simulink model "Demo"  (R2024b)
settings: Solver=FixedStepDiscrete  StartTime=0.0  StopTime=15  FixedStep=0.001  RelTol=1e-3
InitFcn:
  | LCS_parameters
values from neighbouring files (symbols this model uses):
  BREFF = 1.9697    [LCS_parameters.m]
  carMass = 251.54    [LCS_parameters.m]
  CGheight = 0.253    [LCS_parameters.m]
  Cz = 87563    [LCS_parameters.m]
  DREFF = 0.54832    [LCS_parameters.m]
  FNOMIN = 1295    [LCS_parameters.m]
  FREFF = 0.017609    [LCS_parameters.m]
  gearRatio = 13.75    [LCS_parameters.m]
  LONGVL = 10    [LCS_parameters.m]
  nominalWheelRadius = 0.197    [LCS_parameters.m]
  optimalSlipRatio = 0.11    [LCS_parameters.m]
  Q_REO = 1    [LCS_parameters.m]
  Q_V1 = 0.0034187    [LCS_parameters.m]
  ss_error = [88.7600822305642	89.0376071734511	89.3159282635258	89.5955216735338	89.8756411218665	90.1570974487717	90.4395677327939	90.7230274541677	91.0072189085757	91.2921635447457	91.5779490537006	91.8650704841512	92.1538219996540	92.4426633861175	92.7316475908439	93.0233476422096	93.3140548464672	93.6068138765075	93.9008352694172	94.1935963586418	94.4902272246880	94.7850545124692	95.0823324329676	95.38056 ...(+2780 chars)    [LCS_parameters.m]
  unloadedRadius = 0.2032    [LCS_parameters.m]
  wheelbaseLength = 1.53    [LCS_parameters.m]
undefined symbols (not defined in the file or in its folder): dspblkCoreblockFVToolHelper, gcbh
libraries: Solver_SF x1, simulink x1
settings Model: NumberOfSteps=100  Creator=account  LastModifiedBy=xoxi.1

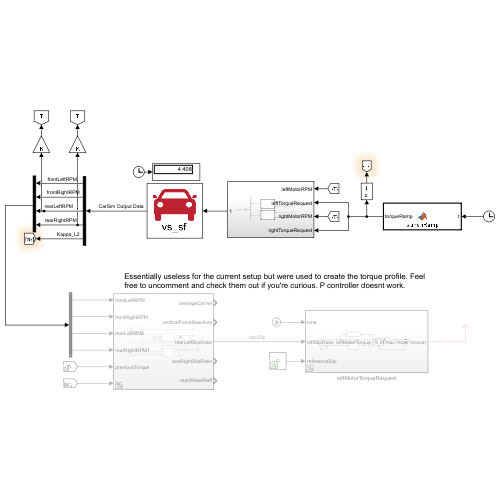
[thumbnail: Simulink's stored preview of the top-level diagram]
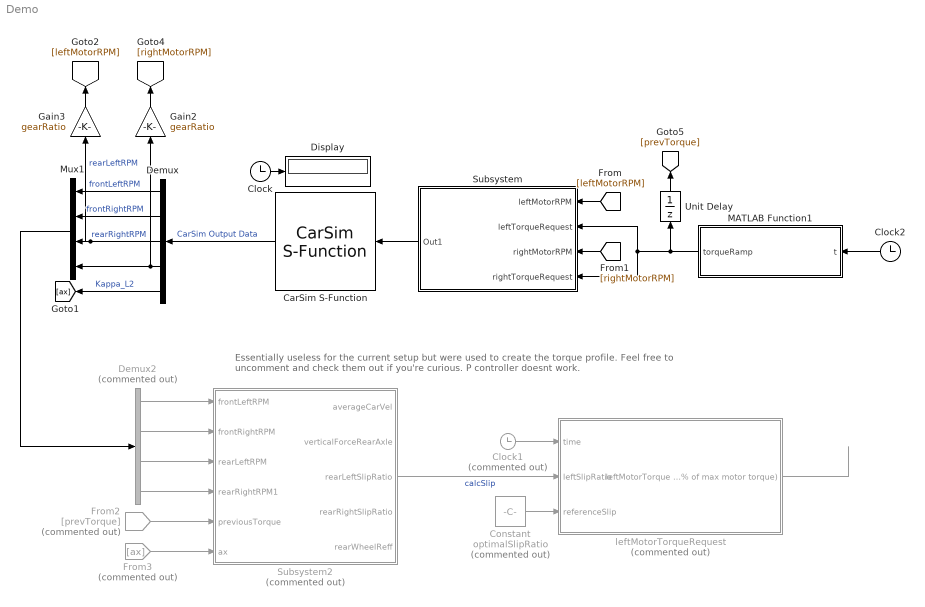
== system Demo ==
  note: Essentially useless for the current setup but were used to create the torque profile. Feel free to uncomment and check them out if you're curious. P controller doesnt work.
  CarSim S-Function : Solver_SF/CarSim S-Function  Priority=1  SIMFILE=simfile.sim  Run_RTs=off  vs_state_ind=Run  StopMode_ind=Vehicle Model
  Clock : Clock
  Clock1 : Clock  Commented=on
  Clock2 : Clock
  Constant : Constant  Commented=on  Value=optimalSlipRatio
  Demux : Demux  Outputs=5
  Demux2 : Demux  Commented=on
  Display : Display
  From2 : From  Commented=on  GotoTag=prevTorque
  From3 : From  Commented=on  GotoTag=ax
  Gain2 : Gain  Gain=gearRatio
  Gain3 : Gain  Gain=gearRatio
  MATLAB Function1 : MATLAB Function  TreatAsAtomicUnit=on
  Mux1 : Mux
  Subsystem : Subsystem
  Subsystem2 : Subsystem  Commented=on
  Unit Delay : UnitDelay  SampleTime=-1  HasFrameUpgradeWarning=on
  leftMotorTorqueRequest : Subsystem  Commented=on
  wires:
  CarSim S-Function/1 -> Demux/1  "CarSim Output Data"
  Demux/1 -> Mux1/1  "frontLeftRPM"
  Demux/2 -> Mux1/2  "frontRightRPM"
  Demux/3 -> Mux1/3, Gain3/1  "rearLeftRPM"
  Mux1/1 -> Demux2/1
  Demux/4 -> Mux1/4, Gain2/1  "rearRightRPM"
  Demux2/1 -> Subsystem2/1(frontLeftRPM)
  Demux2/2 -> Subsystem2/2(frontRightRPM)
  From2/1 -> Subsystem2/5(previousTorque)
  Demux2/4 -> Subsystem2/4(rearRightRPM1)
  Demux2/3 -> Subsystem2/3(rearLeftRPM)
  Subsystem2/3(rearLeftSlipRatio) -> leftMotorTorqueRequest/2(leftSlipRatio)  "calcSlip"
  Clock1/1 -> leftMotorTorqueRequest/1(time)
  Subsystem/1(Out1) -> CarSim S-Function/1
  [leftMotorRPM] -> Subsystem/1(leftMotorRPM)
  [rightMotorRPM] -> Subsystem/3(rightMotorRPM)
  From3/1 -> Subsystem2/6(ax)
  Constant/1 -> leftMotorTorqueRequest/3(referenceSlip)
  MATLAB Function1/1(torqueRamp) -> Subsystem/4(rightTorqueRequest), Subsystem/2(leftTorqueRequest), Unit Delay/1
  Clock2/1 -> MATLAB Function1/1(t)
  Unit Delay/1 -> [prevTorque]
  leftMotorTorqueRequest/1(leftMotorTorque (% of max motor torque)) -> ?
  Clock/1 -> Display/1
  Demux/5 -> [ax]  "Kappa_L2"
  Gain2/1 -> [rightMotorRPM]
  Gain3/1 -> [leftMotorRPM]

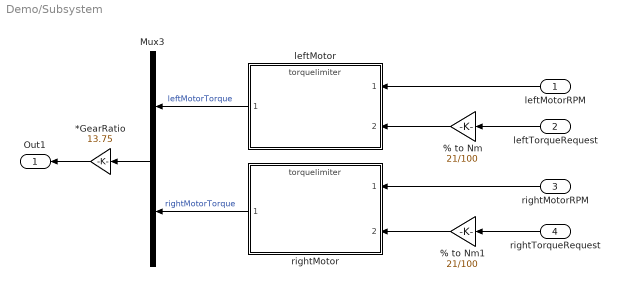
== system Demo/Subsystem ==
  leftMotorRPM : Inport
  leftTorqueRequest : Inport  Port=2
  rightMotorRPM : Inport  Port=3
  rightTorqueRequest : Inport  Port=4
  % to Nm : Gain  Gain=21/100
  % to Nm1 : Gain  Gain=21/100
  *GearRatio : Gain  Gain=13.75
  Mux3 : Mux  Inputs=2
  leftMotor : ModelReference  ModelNameDialog=torquelimiter.slx  SimulationMode=Normal  ModelReferenceVersion=1.5
  rightMotor : ModelReference  ModelNameDialog=torquelimiter.slx  SimulationMode=Normal  ModelReferenceVersion=1.5
  Out1 : Outport
  wires:
  rightMotor/1 -> Mux3/2  "rightMotorTorque"
  *GearRatio/1 -> Out1/1
  Mux3/1 -> *GearRatio/1
  leftMotor/1 -> Mux3/1  "leftMotorTorque"
  rightTorqueRequest/1 -> % to Nm1/1
  leftTorqueRequest/1 -> % to Nm/1
  leftMotorRPM/1 -> leftMotor/1
  rightMotorRPM/1 -> rightMotor/1
  % to Nm/1 -> leftMotor/2
  % to Nm1/1 -> rightMotor/2

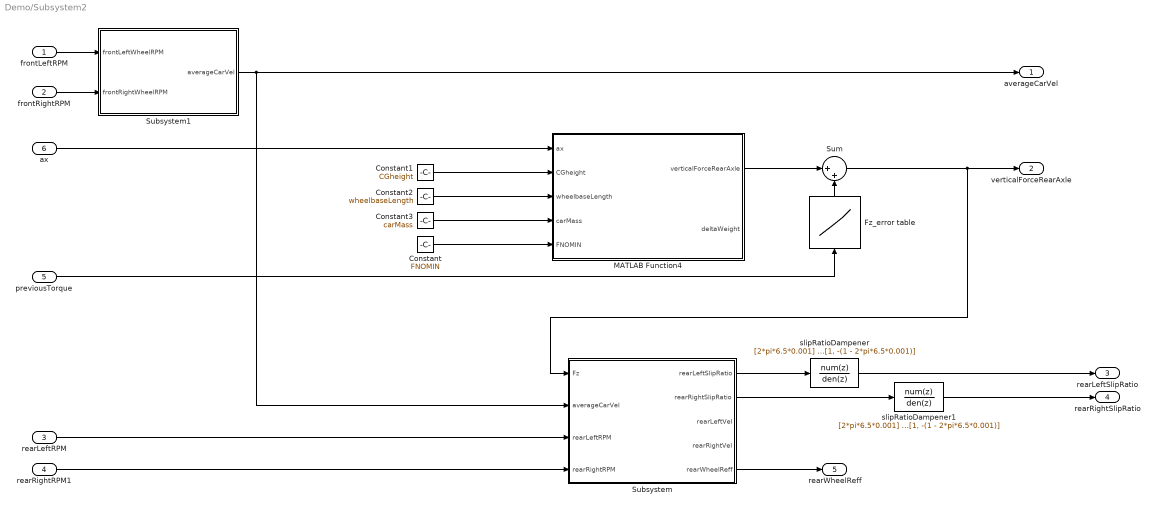
== system Demo/Subsystem2 ==
  frontLeftRPM : Inport
  frontRightRPM : Inport  Port=2
  rearLeftRPM : Inport  Port=3
  rearRightRPM1 : Inport  Port=4
  previousTorque : Inport  Port=5
  ax : Inport  Port=6
  Constant : Constant  Value=FNOMIN
  Constant1 : Constant  Value=CGheight
  Constant2 : Constant  Value=wheelbaseLength
  Constant3 : Constant  Value=carMass
  Fz_error table : Lookup_n-D  NumberOfTableDimensions=1  BreakpointsForDimension1=[7:0.5:100]  Table=ss_error  InternalRulePriority=Speed  RndMeth=Simplest
  MATLAB Function4 : MATLAB Function  TreatAsAtomicUnit=on
  Subsystem : Subsystem
  Subsystem1 : Subsystem
  Sum : Sum  Inputs=|++
  slipRatioDampener : DiscreteTransferFcn  LoadFcn=dspblkCoreblockFVToolHelper(gcbh,'load');  Numerator=[2*pi*6.5*0.001]  Denominator=[1, -(1 - 2*pi*6.5*0.001)]
      settings: CopyFcn=dspblkCoreblockFVToolHelper(gcbh,'copy');  DeleteFcn=dspblkCoreblockFVToolHelper(gcbh,'close');  ModelCloseFcn=dspblkCoreblockFVToolHelper(gcbh,'close');  PreSaveFcn=dspblkCoreblockFVToolHelper(gcbh,'presave');  PostSaveFcn=dspblkCoreblockFVToolHelper(gcbh,'postsave');  CloseFcn=dspblkCoreblockFVToolHelper(gcbh,'close');
  slipRatioDampener1 : DiscreteTransferFcn  LoadFcn=dspblkCoreblockFVToolHelper(gcbh,'load');  Numerator=[2*pi*6.5*0.001]  Denominator=[1, -(1 - 2*pi*6.5*0.001)]
      settings: CopyFcn=dspblkCoreblockFVToolHelper(gcbh,'copy');  DeleteFcn=dspblkCoreblockFVToolHelper(gcbh,'close');  ModelCloseFcn=dspblkCoreblockFVToolHelper(gcbh,'close');  PreSaveFcn=dspblkCoreblockFVToolHelper(gcbh,'presave');  PostSaveFcn=dspblkCoreblockFVToolHelper(gcbh,'postsave');  CloseFcn=dspblkCoreblockFVToolHelper(gcbh,'close');
  averageCarVel : Outport
  verticalForceRearAxle : Outport  Port=2
  rearLeftSlipRatio : Outport  Port=3
  rearRightSlipRatio : Outport  Port=4
  rearWheelReff : Outport  Port=5
  wires:
  frontLeftRPM/1 -> Subsystem1/1(frontLeftWheelRPM)
  Subsystem1/1(averageCarVel) -> averageCarVel/1, Subsystem/2(averageCarVel)
  frontRightRPM/1 -> Subsystem1/2(frontRightWheelRPM)
  Constant3/1 -> MATLAB Function4/4(carMass)
  Constant1/1 -> MATLAB Function4/2(CGheight)
  Constant2/1 -> MATLAB Function4/3(wheelbaseLength)
  previousTorque/1 -> Fz_error table/1
  Sum/1 -> Subsystem/1(Fz), verticalForceRearAxle/1
  Fz_error table/1 -> Sum/2
  Constant/1 -> MATLAB Function4/5(FNOMIN)
  rearLeftRPM/1 -> Subsystem/3(rearLeftRPM)
  rearRightRPM1/1 -> Subsystem/4(rearRightRPM)
  Subsystem/5(rearWheelReff) -> rearWheelReff/1
  MATLAB Function4/1(verticalForceRearAxle) -> Sum/1
  Subsystem/1(rearLeftSlipRatio) -> slipRatioDampener/1
  ax/1 -> MATLAB Function4/1(ax)
  Subsystem/2(rearRightSlipRatio) -> slipRatioDampener1/1
  slipRatioDampener/1 -> rearLeftSlipRatio/1
  slipRatioDampener1/1 -> rearRightSlipRatio/1

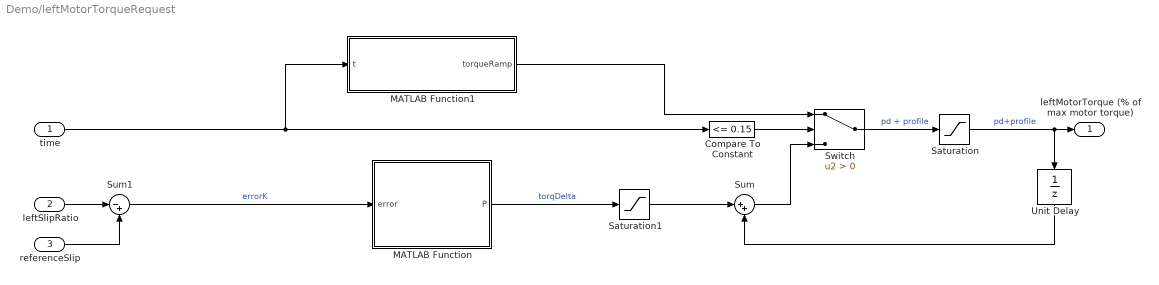
== system Demo/leftMotorTorqueRequest ==
  time : Inport
  leftSlipRatio : Inport  Port=2
  referenceSlip : Inport  Port=3
  Compare To Constant : simulink/Logic and Bit Operations/Compare To Constant  relop=<=  const=0.15  OutDataTypeStr=boolean
  MATLAB Function : MATLAB Function  TreatAsAtomicUnit=on
  MATLAB Function1 : MATLAB Function  TreatAsAtomicUnit=on
  Saturation : Saturate  UpperLimit=100  LowerLimit=0
  Saturation1 : Saturate  UpperLimit=0.05  LowerLimit=-1
  Sum : Sum  Inputs=|++
  Sum1 : Sum  Inputs=|-+
  Switch : Switch  Criteria=u2 > Threshold  SaturateOnIntegerOverflow=off  InputSameDT=off
  Unit Delay : UnitDelay  InitialCondition=30  SampleTime=-1  HasFrameUpgradeWarning=on
  leftMotorTorque (% of max motor torque) : Outport
  wires:
  Switch/1 -> Saturation/1  "pd + profile"
  Compare To Constant/1 -> Switch/2
  time/1 -> MATLAB Function1/1(t), Compare To Constant/1
  referenceSlip/1 -> Sum1/2
  leftSlipRatio/1 -> Sum1/1
  Sum1/1 -> MATLAB Function/1(error)  "errorK"
  Unit Delay/1 -> Sum/2
  Saturation/1 -> Unit Delay/1, leftMotorTorque (% of max motor torque)/1  "pd+profile"
  MATLAB Function1/1(torqueRamp) -> Switch/1
  Sum/1 -> Switch/3
  MATLAB Function/1(P) -> Saturation1/1  "torqDelta"
  Saturation1/1 -> Sum/1

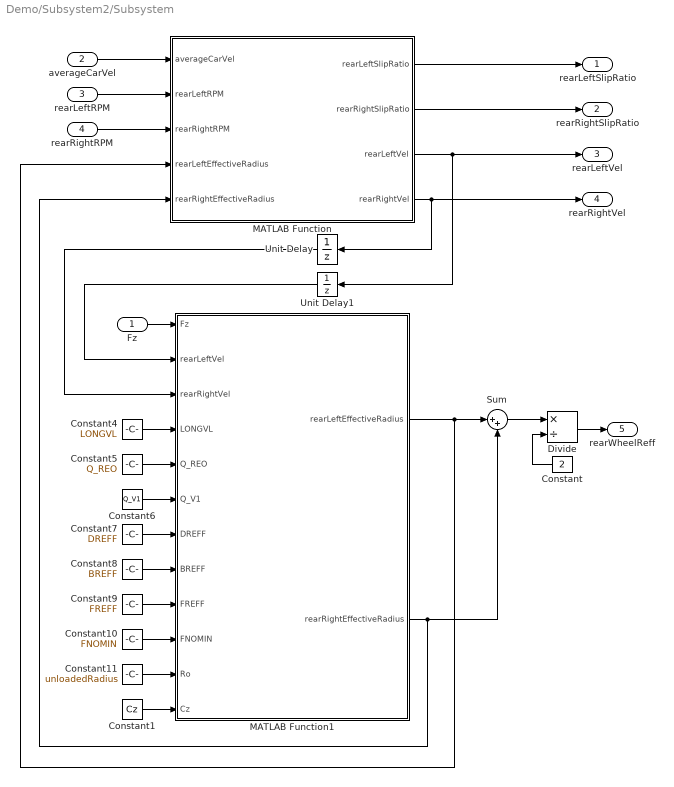
== system Demo/Subsystem2/Subsystem ==
  Fz : Inport
  averageCarVel : Inport  Port=2
  rearLeftRPM : Inport  Port=3
  rearRightRPM : Inport  Port=4
  Constant : Constant  Value=2
  Constant1 : Constant  Value=Cz
  Constant10 : Constant  Value=FNOMIN
  Constant11 : Constant  Value=unloadedRadius
  Constant4 : Constant  Value=LONGVL
  Constant5 : Constant  Value=Q_REO
  Constant6 : Constant  Value=Q_V1
  Constant7 : Constant  Value=DREFF
  Constant8 : Constant  Value=BREFF
  Constant9 : Constant  Value=FREFF
  Divide : Product  Inputs=*/
  MATLAB Function : MATLAB Function  TreatAsAtomicUnit=on
  MATLAB Function1 : MATLAB Function  TreatAsAtomicUnit=on
  Sum : Sum  Inputs=|++
  Unit Delay : UnitDelay  SampleTime=-1  HasFrameUpgradeWarning=on
  Unit Delay1 : UnitDelay  SampleTime=-1  HasFrameUpgradeWarning=on
  rearLeftSlipRatio : Outport
  rearRightSlipRatio : Outport  Port=2
  rearLeftVel : Outport  Port=3
  rearRightVel : Outport  Port=4
  rearWheelReff : Outport  Port=5
  wires:
  Constant8/1 -> MATLAB Function1/8(BREFF)
  MATLAB Function/3(rearLeftVel) -> Unit Delay1/1, rearLeftVel/1
  averageCarVel/1 -> MATLAB Function/1(averageCarVel)
  Unit Delay/1 -> MATLAB Function1/3(rearRightVel)
  Constant4/1 -> MATLAB Function1/4(LONGVL)
  Constant6/1 -> MATLAB Function1/6(Q_V1)
  Constant9/1 -> MATLAB Function1/9(FREFF)
  MATLAB Function1/2(rearRightEffectiveRadius) -> Sum/2, MATLAB Function/5(rearRightEffectiveRadius)
  MATLAB Function/4(rearRightVel) -> rearRightVel/1, Unit Delay/1
  Constant5/1 -> MATLAB Function1/5(Q_REO)
  Fz/1 -> MATLAB Function1/1(Fz)
  Unit Delay1/1 -> MATLAB Function1/2(rearLeftVel)
  Constant7/1 -> MATLAB Function1/7(DREFF)
  Constant10/1 -> MATLAB Function1/10(FNOMIN)
  Constant11/1 -> MATLAB Function1/11(Ro)
  rearLeftRPM/1 -> MATLAB Function/2(rearLeftRPM)
  rearRightRPM/1 -> MATLAB Function/3(rearRightRPM)
  MATLAB Function/2(rearRightSlipRatio) -> rearRightSlipRatio/1
  MATLAB Function/1(rearLeftSlipRatio) -> rearLeftSlipRatio/1
  MATLAB Function1/1(rearLeftEffectiveRadius) -> Sum/1, MATLAB Function/4(rearLeftEffectiveRadius)
  Constant1/1 -> MATLAB Function1/12(Cz)
  Sum/1 -> Divide/1
  Constant/1 -> Divide/2
  Divide/1 -> rearWheelReff/1

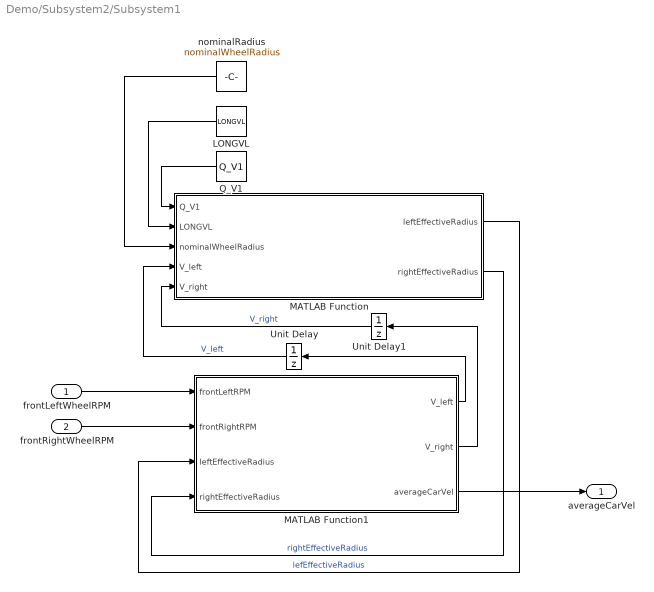
== system Demo/Subsystem2/Subsystem1 ==
  frontLeftWheelRPM : Inport
  frontRightWheelRPM : Inport  Port=2
  LONGVL : Constant  Value=LONGVL
  MATLAB Function : MATLAB Function  TreatAsAtomicUnit=on
  MATLAB Function1 : MATLAB Function  TreatAsAtomicUnit=on
  Q_V1 : Constant  Value=Q_V1
  Unit Delay : UnitDelay  SampleTime=-1  HasFrameUpgradeWarning=on
  Unit Delay1 : UnitDelay  SampleTime=-1  HasFrameUpgradeWarning=on
  nominalRadius : Constant  Value=nominalWheelRadius
  averageCarVel : Outport
  wires:
  frontLeftWheelRPM/1 -> MATLAB Function1/1(frontLeftRPM)
  frontRightWheelRPM/1 -> MATLAB Function1/2(frontRightRPM)
  MATLAB Function1/3(averageCarVel) -> averageCarVel/1
  Q_V1/1 -> MATLAB Function/1(Q_V1)
  LONGVL/1 -> MATLAB Function/2(LONGVL)
  nominalRadius/1 -> MATLAB Function/3(nominalWheelRadius)
  MATLAB Function1/1(V_left) -> Unit Delay/1
  MATLAB Function1/2(V_right) -> Unit Delay1/1
  Unit Delay/1 -> MATLAB Function/4(V_left)  "V_left"
  Unit Delay1/1 -> MATLAB Function/5(V_right)  "V_right"
  MATLAB Function/1(leftEffectiveRadius) -> MATLAB Function1/3(leftEffectiveRadius)  "lefEffectiveRadius"
  MATLAB Function/2(rightEffectiveRadius) -> MATLAB Function1/4(rightEffectiveRadius)  "rightEffectiveRadius"

== matlab function Demo/MATLAB Function1 ==
  data: t input; torqueRamp output
function torqueRamp = launchRamp(t)
  if t <= 1.0
      torqueRamp = -295.875*t^4 + 816.75*t^3 - 798.125*t^2 + 329.5*t + 33.75;
elseif t <= 2.0
      s = t - 1.0;
      torqueRamp = -1.185185185*s^4 + (-14.81481481)*s^3 + 28.51851852*s^2 + (-3.518518519)*s + 86;
elseif t <= 2.4
      s = t - 2.0;
      torqueRamp = -156.25*s^3 + 93.75*s^2 + 95;
else
      torqueRamp = 100;
end
  torqueRamp = min(max(torqueRamp, 0), 100);
end

== matlab function Demo/leftMotorTorqueRequest/MATLAB Function ==
  data: error input; P output
function P = calcP(error)
kP_up = 10;
kP_down = 10;
    if error >= 0
        P = kP_up * error;
        P = min(P, 5);
    else
        P = kP_down * error;
        P = max(P, -25);
    end
end

== matlab function Demo/leftMotorTorqueRequest/MATLAB Function1 ==
  data: t input; torqueRamp output
function torqueRamp = launchRamp(t)
    if t <= 0.05
        s = t - 0.00;
        torqueRamp = 1186.4286*s - 74571.4286*s^3;
    elseif t <= 0.10
        s = t - 0.05;
        torqueRamp = 50 + 627.1429*s - 11185.7143*s^2 + 84857.1429*s^3;
    elseif t <= 0.15
        s = t - 0.10;
        torqueRamp = 64 + 145.0000*s + 1542.8571*s^2 - 16857.1429*s^3;
    elseif t <= 0.20
        s = t - 0.15;
        torqueRamp = 73 + 172.8571*s - 985.7143*s^2 + 6571.4286*s^3;
    else
        torqueRamp = 80;
    end
    torqueRamp = min(max(torqueRamp, 0), 100);
end

== matlab function Demo/Subsystem2/Subsystem1/MATLAB Function ==
  data: Q_V1 input; leftEffectiveRadius output; LONGVL input; nominalWheelRadius input; V_left input; rightEffectiveRadius output; V_right input
function [leftEffectiveRadius, rightEffectiveRadius] = calculateEffectiveRadius(Q_V1, LONGVL, nominalWheelRadius, V_left, V_right)

leftEffectiveRadius = nominalWheelRadius * (1 + Q_V1 * (V_left / LONGVL)^2);
rightEffectiveRadius = nominalWheelRadius * (1 + Q_V1 * (V_right / LONGVL)^2);

end

== matlab function Demo/Subsystem2/Subsystem1/MATLAB Function1 ==
  data: V_left output; V_right output; frontLeftRPM input; averageCarVel output; frontRightRPM input; leftEffectiveRadius input; rightEffectiveRadius input
function [V_left, V_right, averageCarVel] = caclVelwithRealRe(frontLeftRPM, frontRightRPM, leftEffectiveRadius, rightEffectiveRadius)

V_left = leftEffectiveRadius * (frontLeftRPM * 2*pi/60);
V_right = rightEffectiveRadius * (frontRightRPM * 2*pi/60);

averageCarVel = (V_left+V_right)/2;

end

== matlab function Demo/Subsystem2/MATLAB Function4 ==
  data: ax input; CGheight input; wheelbaseLength input; carMass input; verticalForceRearAxle output; deltaWeight output; FNOMIN input
function [verticalForceRearAxle, deltaWeight] = calcVerticalForce(ax, CGheight, wheelbaseLength, carMass, FNOMIN)

deltaWeight = (carMass * ax * CGheight) / wheelbaseLength;

verticalForceRearAxle = FNOMIN + deltaWeight;

end

== matlab function Demo/Subsystem2/Subsystem/MATLAB Function ==
  data: rearLeftSlipRatio output; rearRightSlipRatio output; averageCarVel input; rearLeftRPM input; rearLeftVel output; rearRightRPM input; rearLeftEffectiveRadius input; rearRightEffectiveRadius input; rearRightVel output
function [rearLeftSlipRatio, rearRightSlipRatio, rearLeftVel, rearRightVel] = calculateRearVel(averageCarVel, rearLeftRPM, rearRightRPM, rearLeftEffectiveRadius, rearRightEffectiveRadius)

rearLeftVel = rearLeftEffectiveRadius * (rearLeftRPM * 2*pi/60);
rearRightVel = rearRightEffectiveRadius * (rearRightRPM * 2*pi/60);

rearLeftSlipRatio = (rearLeftVel/averageCarVel) - 1 -0.005;
rearRightSlipRatio = (rearRightVel/averageCarVel) - 1 - 0.005;
end

== matlab function Demo/Subsystem2/Subsystem/MATLAB Function1 ==
  data: Fz input; rearLeftVel input; rearLeftEffectiveRadius output; rearRightVel input; LONGVL input; Q_REO input; Q_V1 input; DREFF input; BREFF input; FREFF input; FNOMIN input; Ro input; rearRightEffectiveRadius output; Cz input
function [rearLeftEffectiveRadius, rearRightEffectiveRadius] = calculateRearEffectiveRadius(Fz, rearLeftVel, rearRightVel, LONGVL, Q_REO, Q_V1, DREFF, BREFF, FREFF, FNOMIN, Ro, Cz)
    
    Fz = Fz / 2;  % split total axle load equally per wheel
    
    rearLeftRomega  = Ro * (Q_REO + Q_V1 * (rearLeftVel  / LONGVL)^2);
    rearRightRomega = Ro * (Q_REO + Q_V1 * (rearRightVel / LONGVL)^2);
    
    rearLeftEffectiveRadius  = rearLeftRomega  - (Fz / Cz) * (DREFF * atan(BREFF * Fz / FNOMIN) + FREFF * Fz / FNOMIN);
    rearRightEffectiveRadius = rearRightRomega - (Fz / Cz) * (DREFF * atan(BREFF * Fz / FNOMIN) + FREFF * Fz / FNOMIN);

    rearLeftEffectiveRadius = rearLeftEffectiveRadius - 0.0025;
    rearRightEffectiveRadius = rearRightEffectiveRadius - 0.0025;

end
